simulink subsystem "bh_COMPONENT_3LINK_hand_Newton"  (R2022b)
settings: Solver=VariableStepAuto  StartTime=0.0  StopTime=10.0  RelTol=1e-3
undefined symbols (not defined in the file): IC, robo_params
settings Model: Creator=bhorton  LastModifiedBy=bhorton
settings SolverCC: AlgebraicLoopSolver=TrustRegion
settings DebuggingCC: UnconnectedInputMsg=warning  UnconnectedOutputMsg=warning  UnconnectedLineMsg=warning  SFMachineParentedDataDiag=warning
settings ModelReferenceCC: EnableRefExpFcnMdlSchedulingChecks=on
settings RTWCC: DLArmComputeVersion=19.05

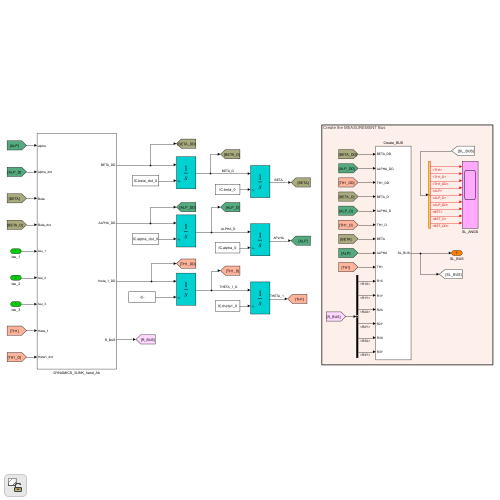
[thumbnail: Simulink's stored preview of the top-level diagram]
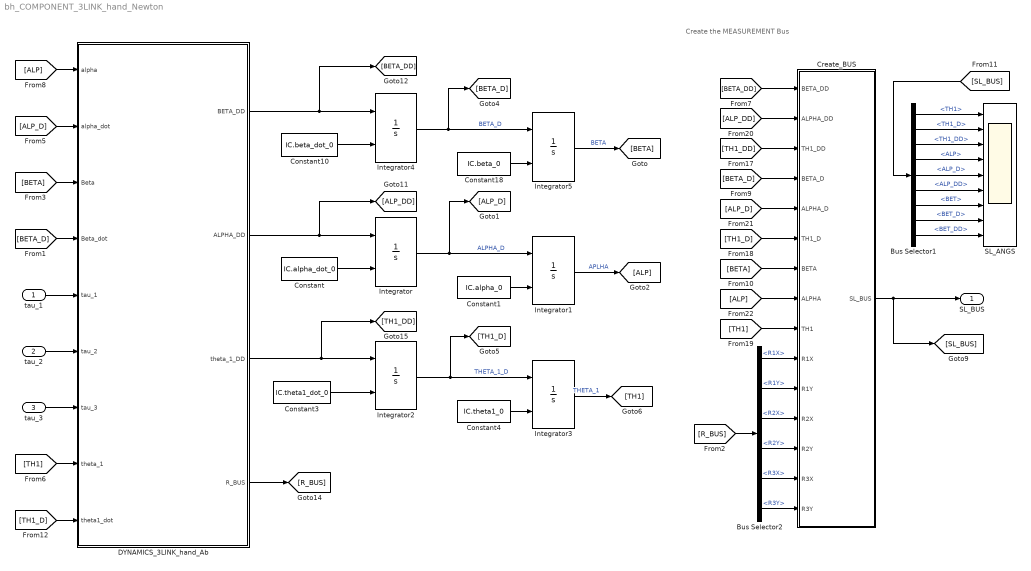
== system bh_COMPONENT_3LINK_hand_Newton ==
  note: Create the MEASUREMENT Bus
  tau_1 : Inport
  tau_2 : Inport  Port=2
  tau_3 : Inport  Port=3
  Bus Selector1 : BusSelector  OutputSignals=TH1,TH1_D,TH1_DD,ALP,ALP_D,ALP_DD,BET,BET_D,BET_DD
  Bus Selector2 : BusSelector  OutputSignals=R1X,R1Y,R2X,R2Y,R3X,R3Y
  Constant : Constant  Value=IC.alpha_dot_0
  Constant1 : Constant  Value=IC.alpha_0
  Constant10 : Constant  Value=IC.beta_dot_0
  Constant18 : Constant  Value=IC.beta_0
  Constant3 : Constant  Value=IC.theta1_dot_0
  Constant4 : Constant  Value=IC.theta1_0
  Create_BUS : Subsystem
  DYNAMICS_3LINK_hand_Ab : Subsystem
  Integrator{,1..5} (6 alike) : Integrator  InitialConditionSource=external
  SL_ANGS : Scope  NumInputPorts=9
  SL_BUS : Outport
  wires:
  Create_BUS/1(SL_BUS) -> SL_BUS/1, [SL_BUS]
  Bus Selector1/7 -> SL_ANGS/7  "<BET>"
  Bus Selector1/1 -> SL_ANGS/1  "<TH1>"
  [R_BUS] -> Bus Selector2/1
  [TH1] -> DYNAMICS_3LINK_hand_Ab/8(theta_1)
  DYNAMICS_3LINK_hand_Ab/4(R_BUS) -> [R_BUS]
  Bus Selector1/4 -> SL_ANGS/4  "<ALP>"
  [TH1_D] -> DYNAMICS_3LINK_hand_Ab/9(theta1_dot)
  tau_2/1 -> DYNAMICS_3LINK_hand_Ab/6(tau_2)
  Bus Selector1/3 -> SL_ANGS/3  "<TH1_DD>"
  Bus Selector2/1 -> Create_BUS/10(R1X)  "<R1X>"
  tau_3/1 -> DYNAMICS_3LINK_hand_Ab/7(tau_3)
  Bus Selector1/6 -> SL_ANGS/6  "<ALP_DD>"
  Bus Selector2/2 -> Create_BUS/11(R1Y)  "<R1Y>"
  DYNAMICS_3LINK_hand_Ab/2(ALPHA_DD) -> [ALP_DD], Integrator/1
  Constant1/1 -> Integrator1/2
  [BETA] -> DYNAMICS_3LINK_hand_Ab/3(Beta)
  tau_1/1 -> DYNAMICS_3LINK_hand_Ab/5(tau_1)
  [BETA_D] -> DYNAMICS_3LINK_hand_Ab/4(Beta_dot)
  [ALP] -> Create_BUS/8(ALPHA)
  [ALP] -> DYNAMICS_3LINK_hand_Ab/1(alpha)
  DYNAMICS_3LINK_hand_Ab/3(theta_1_DD) -> [TH1_DD], Integrator2/1
  [TH1_DD] -> Create_BUS/3(TH1_DD)
  [SL_BUS] -> Bus Selector1/1
  [BETA_D] -> Create_BUS/4(BETA_D)
  Bus Selector1/2 -> SL_ANGS/2  "<TH1_D>"
  Bus Selector1/5 -> SL_ANGS/5  "<ALP_D>"
  [BETA] -> Create_BUS/7(BETA)
  [ALP_DD] -> Create_BUS/2(ALPHA_DD)
  [BETA_DD] -> Create_BUS/1(BETA_DD)
  Bus Selector1/8 -> SL_ANGS/8  "<BET_D>"
  Constant18/1 -> Integrator5/2
  [ALP_D] -> Create_BUS/5(ALPHA_D)
  Integrator5/1 -> [BETA]  "BETA"
  [TH1] -> Create_BUS/9(TH1)
  DYNAMICS_3LINK_hand_Ab/1(BETA_DD) -> [BETA_DD], Integrator4/1
  Constant/1 -> Integrator/2
  Integrator2/1 -> [TH1_D], Integrator3/1  "THETA_1_D"
  Integrator4/1 -> [BETA_D], Integrator5/1  "BETA_D"
  Integrator1/1 -> [ALP]  "APLHA"
  Constant10/1 -> Integrator4/2
  Bus Selector1/9 -> SL_ANGS/9  "<BET_DD>"
  [TH1_D] -> Create_BUS/6(TH1_D)
  Integrator/1 -> [ALP_D], Integrator1/1  "ALPHA_D"
  [ALP_D] -> DYNAMICS_3LINK_hand_Ab/2(alpha_dot)
  Constant3/1 -> Integrator2/2
  Constant4/1 -> Integrator3/2
  Integrator3/1 -> [TH1]  "THETA_1"
  Bus Selector2/3 -> Create_BUS/12(R2X)  "<R2X>"
  Bus Selector2/4 -> Create_BUS/13(R2Y)  "<R2Y>"
  Bus Selector2/5 -> Create_BUS/14(R3X)  "<R3X>"
  Bus Selector2/6 -> Create_BUS/15(R3Y)  "<R3Y>"

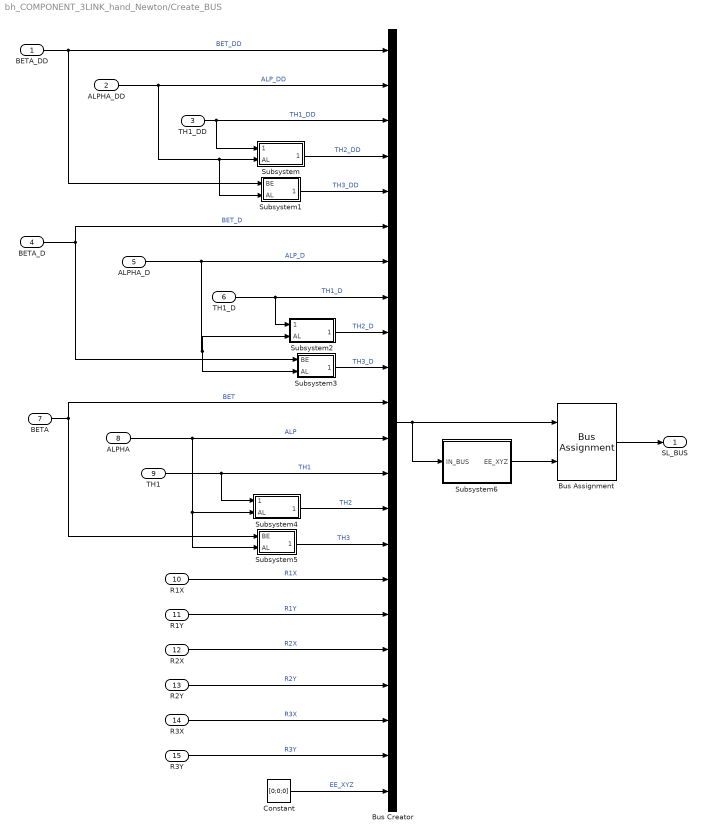
== system bh_COMPONENT_3LINK_hand_Newton/Create_BUS ==
  BETA_DD : Inport
  ALPHA_DD : Inport  Port=2
  TH1_DD : Inport  Port=3
  BETA_D : Inport  Port=4
  ALPHA_D : Inport  Port=5
  TH1_D : Inport  Port=6
  BETA : Inport  Port=7
  ALPHA : Inport  Port=8
  TH1 : Inport  Port=9
  R1X : Inport  Port=10
  R1Y : Inport  Port=11
  R2X : Inport  Port=12
  R2Y : Inport  Port=13
  R3X : Inport  Port=14
  R3Y : Inport  Port=15
  Bus Assignment : BusAssignment  AssignedSignals=EE_XYZ
  Bus Creator : BusCreator  Inputs=22
  Constant : Constant  Value=[0;0;0]
  Subsystem : Subsystem
  Subsystem1 : Subsystem
  Subsystem2 : Subsystem
  Subsystem3 : Subsystem
  Subsystem4 : Subsystem
  Subsystem5 : Subsystem
  Subsystem6 : Subsystem
  SL_BUS : Outport
  wires:
  BETA_DD/1 -> Subsystem1/1(BE), Bus Creator/1  "BET_DD"
  ALPHA_DD/1 -> Bus Creator/2, Subsystem1/2(AL), Subsystem/2(AL)  "ALP_DD"
  TH1_DD/1 -> Subsystem/1(TH_1), Bus Creator/3  "TH1_DD"
  Subsystem/1(TH_2) -> Bus Creator/4  "TH2_DD"
  Subsystem1/1(TH_3) -> Bus Creator/5  "TH3_DD"
  BETA_D/1 -> Subsystem3/1(BE), Bus Creator/6  "BET_D"
  ALPHA_D/1 -> Subsystem3/2(AL), Subsystem2/2(AL), Bus Creator/7  "ALP_D"
  TH1_D/1 -> Subsystem2/1(TH_1), Bus Creator/8  "TH1_D"
  Subsystem2/1(TH_2) -> Bus Creator/9  "TH2_D"
  Subsystem3/1(TH_3) -> Bus Creator/10  "TH3_D"
  BETA/1 -> Subsystem5/1(BE), Bus Creator/11  "BET"
  ALPHA/1 -> Subsystem5/2(AL), Subsystem4/2(AL), Bus Creator/12  "ALP"
  TH1/1 -> Subsystem4/1(TH_1), Bus Creator/13  "TH1"
  Subsystem4/1(TH_2) -> Bus Creator/14  "TH2"
  Subsystem5/1(TH_3) -> Bus Creator/15  "TH3"
  R1X/1 -> Bus Creator/16  "R1X"
  R1Y/1 -> Bus Creator/17  "R1Y"
  R2X/1 -> Bus Creator/18  "R2X"
  R2Y/1 -> Bus Creator/19  "R2Y"
  R3X/1 -> Bus Creator/20  "R3X"
  R3Y/1 -> Bus Creator/21  "R3Y"
  Constant/1 -> Bus Creator/22  "EE_XYZ"
  Bus Creator/1 -> Subsystem6/1(IN_BUS), Bus Assignment/1
  Subsystem6/1(EE_XYZ) -> Bus Assignment/2
  Bus Assignment/1 -> SL_BUS/1

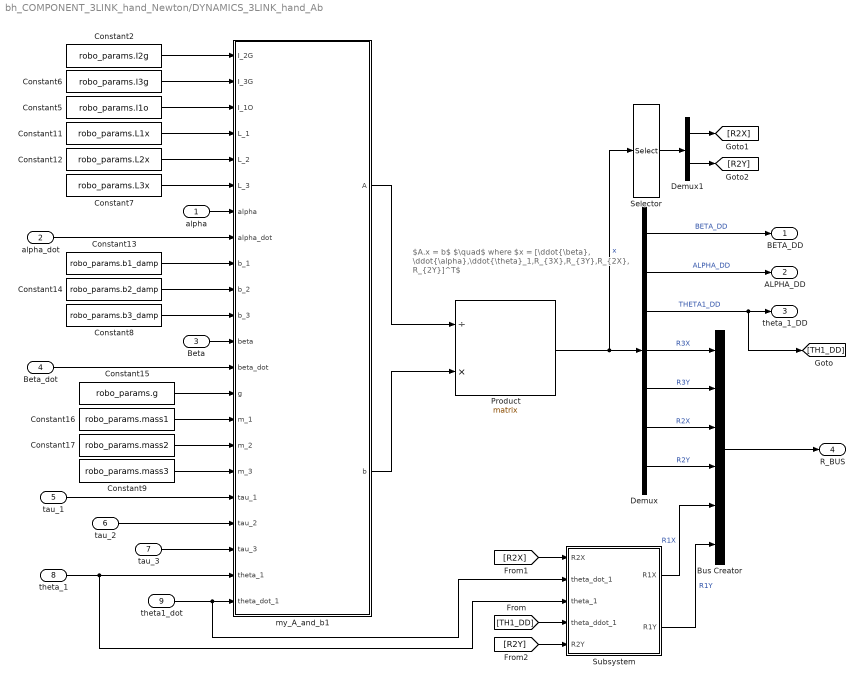
== system bh_COMPONENT_3LINK_hand_Newton/DYNAMICS_3LINK_hand_Ab ==
  note: $A.x = b$ $\quad$ where
      |
      | $x = [\ddot{\beta}, \ddot{\alpha},\ddot{\theta}_1,R_{3X},R_{3Y},R_{2X}, R_{2Y}]^T$
  alpha : Inport
  alpha_dot : Inport  Port=2
  Beta : Inport  Port=3
  Beta_dot : Inport  Port=4
  tau_1 : Inport  Port=5
  tau_2 : Inport  Port=6
  tau_3 : Inport  Port=7
  theta_1 : Inport  Port=8
  theta1_dot : Inport  Port=9
  Bus Creator : BusCreator  Inputs=6
  Constant11 : Constant  Value=robo_params.L1x
  Constant12 : Constant  Value=robo_params.L2x
  Constant13 : Constant  Value=robo_params.b1_damp
  Constant14 : Constant  Value=robo_params.b2_damp
  Constant15 : Constant  Value=robo_params.g
  Constant16 : Constant  Value=robo_params.mass1
  Constant17 : Constant  Value=robo_params.mass2
  Constant2 : Constant  Value=robo_params.I2g
  Constant5 : Constant  Value=robo_params.I1o
  Constant6 : Constant  Value=robo_params.I3g
  Constant7 : Constant  Value=robo_params.L3x
  Constant8 : Constant  Value=robo_params.b3_damp
  Constant9 : Constant  Value=robo_params.mass3
  Demux : Demux  Outputs=7
  Demux1 : Demux  Outputs=2
  Product : Product  Inputs=/*  Multiplication=Matrix(*)
  Selector : Selector  InputPortWidth=7  IndexOptions=Index vector (dialog)  Indices=[6 7]  OutputSizes=1
  Subsystem : Subsystem
  my_A_and_b1 : MATLAB Function  TreatAsAtomicUnit=on
  BETA_DD : Outport
  ALPHA_DD : Outport  Port=2
  theta_1_DD : Outport  Port=3
  R_BUS : Outport  Port=4
  wires:
  Bus Creator/1 -> R_BUS/1
  tau_1/1 -> my_A_and_b1/18(tau_1)
  Demux/2 -> ALPHA_DD/1  "ALPHA_DD"
  Subsystem/2(R1Y) -> Bus Creator/6  "R1Y"
  Demux/4 -> Bus Creator/1  "R3X"
  Constant14/1 -> my_A_and_b1/10(b_2)
  Demux/7 -> Bus Creator/4  "R2Y"
  Demux/1 -> BETA_DD/1  "BETA_DD"
  Subsystem/1(R1X) -> Bus Creator/5  "R1X"
  Constant9/1 -> my_A_and_b1/17(m_3)
  [R2Y] -> Subsystem/5(R2Y)
  Product/1 -> Demux/1, Selector/1  "x"
  alpha/1 -> my_A_and_b1/7(alpha)
  Constant5/1 -> my_A_and_b1/3(I_1O)
  Constant2/1 -> my_A_and_b1/1(I_2G)
  Constant12/1 -> my_A_and_b1/5(L_2)
  theta_1/1 -> my_A_and_b1/21(theta_1), Subsystem/3(theta_1)
  [TH1_DD] -> Subsystem/4(theta_ddot_1)
  Constant15/1 -> my_A_and_b1/14(g)
  Constant13/1 -> my_A_and_b1/9(b_1)
  alpha_dot/1 -> my_A_and_b1/8(alpha_dot)
  Demux/3 -> theta_1_DD/1, [TH1_DD]  "THETA1_DD"
  my_A_and_b1/1(A) -> Product/1
  tau_3/1 -> my_A_and_b1/20(tau_3)
  tau_2/1 -> my_A_and_b1/19(tau_2)
  Constant17/1 -> my_A_and_b1/16(m_2)
  [R2X] -> Subsystem/1(R2X)
  Demux/6 -> Bus Creator/3  "R2X"
  Constant6/1 -> my_A_and_b1/2(I_3G)
  Demux1/2 -> [R2Y]
  Demux/5 -> Bus Creator/2  "R3Y"
  my_A_and_b1/2(b) -> Product/2
  Demux1/1 -> [R2X]
  Beta/1 -> my_A_and_b1/12(beta)
  theta1_dot/1 -> my_A_and_b1/22(theta_dot_1), Subsystem/2(theta_dot_1)
  Beta_dot/1 -> my_A_and_b1/13(beta_dot)
  Constant11/1 -> my_A_and_b1/4(L_1)
  Selector/1 -> Demux1/1
  Constant7/1 -> my_A_and_b1/6(L_3)
  Constant8/1 -> my_A_and_b1/11(b_3)
  Constant16/1 -> my_A_and_b1/15(m_1)

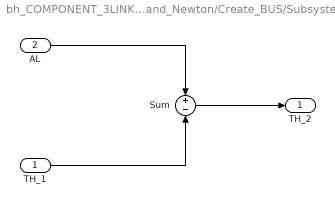
== system bh_COMPONENT_3LINK_hand_Newton/Create_BUS/Subsystem ==
  TH_1 : Inport
  AL : Inport  Port=2
  Sum : Sum  Inputs=+|-
  TH_2 : Outport
  wires:
  Sum/1 -> TH_2/1
  AL/1 -> Sum/1
  TH_1/1 -> Sum/2

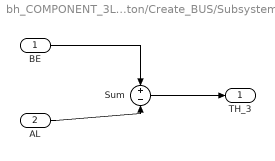
== system bh_COMPONENT_3LINK_hand_Newton/Create_BUS/Subsystem1 ==
  BE : Inport
  AL : Inport  Port=2
  Sum : Sum  Inputs=+|-
  TH_3 : Outport
  wires:
  BE/1 -> Sum/1
  AL/1 -> Sum/2
  Sum/1 -> TH_3/1

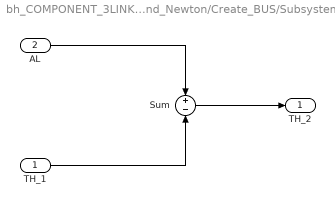
== system bh_COMPONENT_3LINK_hand_Newton/Create_BUS/Subsystem2 ==
  TH_1 : Inport
  AL : Inport  Port=2
  Sum : Sum  Inputs=+|-
  TH_2 : Outport
  wires:
  Sum/1 -> TH_2/1
  AL/1 -> Sum/1
  TH_1/1 -> Sum/2

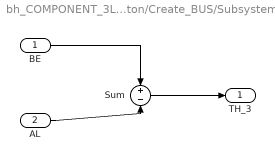
== system bh_COMPONENT_3LINK_hand_Newton/Create_BUS/Subsystem3 ==
  BE : Inport
  AL : Inport  Port=2
  Sum : Sum  Inputs=+|-
  TH_3 : Outport
  wires:
  BE/1 -> Sum/1
  AL/1 -> Sum/2
  Sum/1 -> TH_3/1

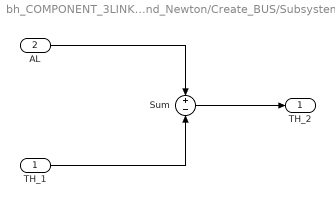
== system bh_COMPONENT_3LINK_hand_Newton/Create_BUS/Subsystem4 ==
  TH_1 : Inport
  AL : Inport  Port=2
  Sum : Sum  Inputs=+|-
  TH_2 : Outport
  wires:
  Sum/1 -> TH_2/1
  AL/1 -> Sum/1
  TH_1/1 -> Sum/2

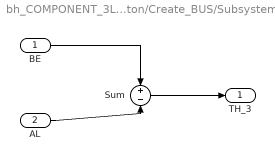
== system bh_COMPONENT_3LINK_hand_Newton/Create_BUS/Subsystem5 ==
  BE : Inport
  AL : Inport  Port=2
  Sum : Sum  Inputs=+|-
  TH_3 : Outport
  wires:
  BE/1 -> Sum/1
  AL/1 -> Sum/2
  Sum/1 -> TH_3/1

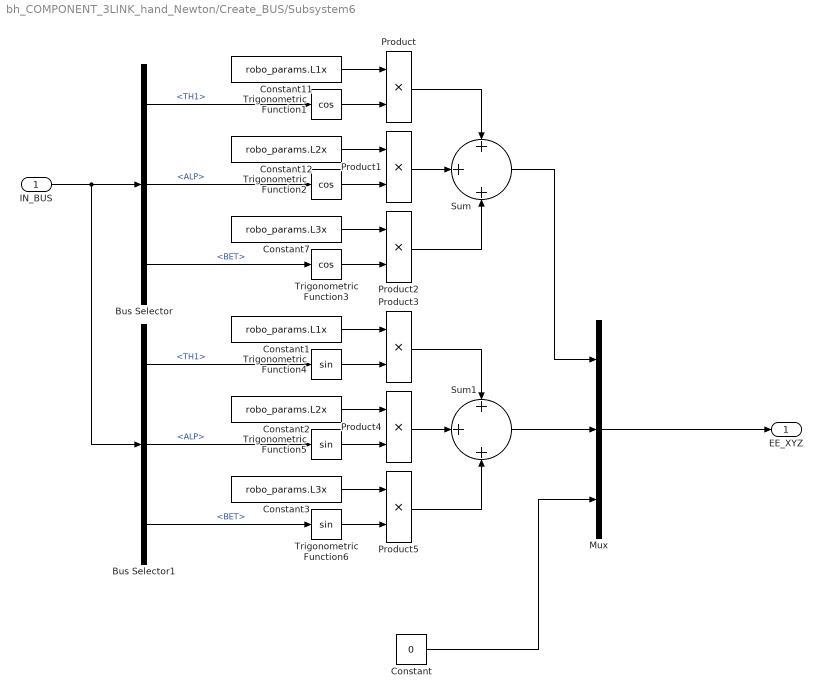
== system bh_COMPONENT_3LINK_hand_Newton/Create_BUS/Subsystem6 ==
  IN_BUS : Inport
  Bus Selector : BusSelector  OutputSignals=TH1,ALP,BET
  Bus Selector1 : BusSelector  OutputSignals=TH1,ALP,BET
  Constant : Constant  Value=0
  Constant1 : Constant  Value=robo_params.L1x
  Constant11 : Constant  Value=robo_params.L1x
  Constant12 : Constant  Value=robo_params.L2x
  Constant2 : Constant  Value=robo_params.L2x
  Constant3 : Constant  Value=robo_params.L3x
  Constant7 : Constant  Value=robo_params.L3x
  Mux : Mux  Inputs=3
  Product{,1..5} (6 alike) : Product
  Sum : Sum  Inputs=+|+|+
  Sum1 : Sum  Inputs=+|+|+
  Trigonometric Function1 : Trigonometry  Operator=cos
  Trigonometric Function2 : Trigonometry  Operator=cos
  Trigonometric Function3 : Trigonometry  Operator=cos
  Trigonometric Function4 : Trigonometry
  Trigonometric Function5 : Trigonometry
  Trigonometric Function6 : Trigonometry
  EE_XYZ : Outport
  wires:
  Bus Selector/1 -> Trigonometric Function1/1  "<TH1>"
  Bus Selector/2 -> Trigonometric Function2/1  "<ALP>"
  Bus Selector/3 -> Trigonometric Function3/1  "<BET>"
  Trigonometric Function1/1 -> Product/2
  Constant11/1 -> Product/1
  Trigonometric Function2/1 -> Product1/2
  Constant12/1 -> Product1/1
  Trigonometric Function3/1 -> Product2/2
  Constant7/1 -> Product2/1
  Product1/1 -> Sum/2
  Product/1 -> Sum/1
  Product2/1 -> Sum/3
  Bus Selector1/3 -> Trigonometric Function6/1  "<BET>"
  Bus Selector1/2 -> Trigonometric Function5/1  "<ALP>"
  Constant1/1 -> Product3/1
  IN_BUS/1 -> Bus Selector1/1, Bus Selector/1
  Bus Selector1/1 -> Trigonometric Function4/1  "<TH1>"
  Constant3/1 -> Product5/1
  Product5/1 -> Sum1/3
  Trigonometric Function6/1 -> Product5/2
  Trigonometric Function4/1 -> Product3/2
  Product3/1 -> Sum1/1
  Trigonometric Function5/1 -> Product4/2
  Constant2/1 -> Product4/1
  Product4/1 -> Sum1/2
  Sum/1 -> Mux/1
  Constant/1 -> Mux/3
  Sum1/1 -> Mux/2
  Mux/1 -> EE_XYZ/1

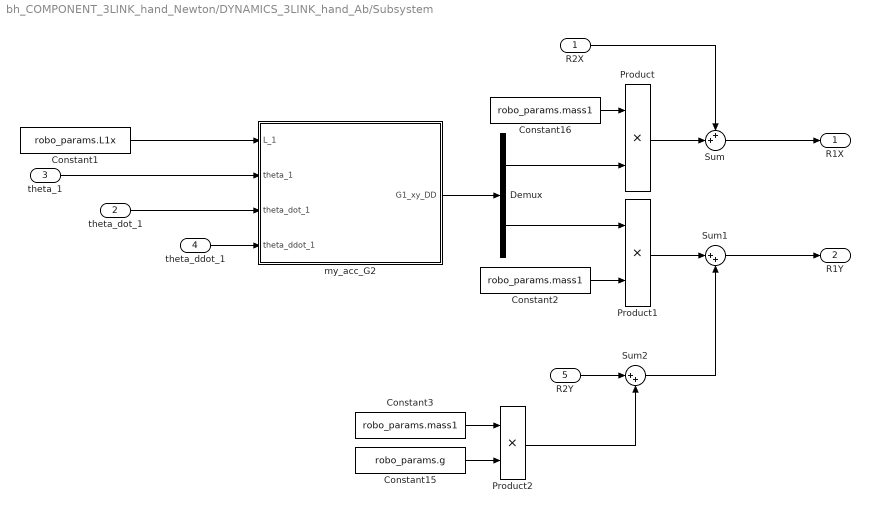
== system bh_COMPONENT_3LINK_hand_Newton/DYNAMICS_3LINK_hand_Ab/Subsystem ==
  R2X : Inport
  theta_dot_1 : Inport  Port=2
  theta_1 : Inport  Port=3
  theta_ddot_1 : Inport  Port=4
  R2Y : Inport  Port=5
  Constant1 : Constant  Value=robo_params.L1x
  Constant15 : Constant  Value=robo_params.g
  Constant16 : Constant  Value=robo_params.mass1
  Constant2 : Constant  Value=robo_params.mass1
  Constant3 : Constant  Value=robo_params.mass1
  Demux : Demux  Outputs=2
  Product : Product
  Product1 : Product
  Product2 : Product
  Sum : Sum  Inputs=++|
  Sum1 : Sum  Inputs=|++
  Sum2 : Sum  Inputs=|++
  my_acc_G2 : MATLAB Function  TreatAsAtomicUnit=on
  R1X : Outport
  R1Y : Outport  Port=2
  wires:
  R2Y/1 -> Sum2/1
  R2X/1 -> Sum/1
  Product2/1 -> Sum2/2
  Constant15/1 -> Product2/2
  Constant3/1 -> Product2/1
  Sum/1 -> R1X/1
  Sum1/1 -> R1Y/1
  Sum2/1 -> Sum1/2
  Product1/1 -> Sum1/1
  Constant2/1 -> Product1/2
  Demux/2 -> Product1/1
  Product/1 -> Sum/2
  Constant16/1 -> Product/1
  Demux/1 -> Product/2
  my_acc_G2/1(G1_xy_DD) -> Demux/1
  theta_dot_1/1 -> my_acc_G2/3(theta_dot_1)
  Constant1/1 -> my_acc_G2/1(L_1)
  theta_1/1 -> my_acc_G2/2(theta_1)
  theta_ddot_1/1 -> my_acc_G2/4(theta_ddot_1)

== matlab function bh_COMPONENT_3LINK_hand_Newton/DYNAMICS_3LINK_hand_Ab/my_A_and_b1 ==
  data: I_2G input; A output; I_3G input; I_1O input; L_1 input; L_2 input; L_3 input; alpha input; alpha_dot input; b_1 input; b_2 input; b_3 input; beta input; beta_dot input; g input; m_1 input; m_2 input; m_3 input; tau_1 input; tau_2 input; tau_3 input; theta_1 input; theta_dot_1 input; b output
function [A,b] = my_A_and_b(I_2G,I_3G,I_1O,L_1,L_2,L_3,alpha,alpha_dot,b_1,b_2,b_3,beta,beta_dot,g,m_1,m_2,m_3,tau_1,tau_2,tau_3,theta_1,theta_dot_1)
%#codegen

%    This function was generated by the Symbolic Math Toolbox version 9.2.
%    28-Oct-2022 10:28:51

A = reshape([L_3.*m_3.*sin(beta).*(-1.0./2.0),(L_3.*m_3.*cos(beta))./2.0,I_3G,0.0,0.0,0.0,0.0,-L_2.*m_3.*sin(alpha),L_2.*m_3.*cos(alpha),0.0,L_2.*m_2.*sin(alpha).*(-1.0./2.0),(L_2.*m_2.*cos(alpha))./2.0,I_2G,0.0,-L_1.*m_3.*sin(theta_1),L_1.*m_3.*cos(theta_1),0.0,-L_1.*m_2.*sin(theta_1),L_1.*m_2.*cos(theta_1),0.0,I_1O,-1.0,0.0,L_3.*sin(beta).*(-1.0./2.0),1.0,0.0,L_2.*sin(alpha).*(-1.0./2.0),0.0,0.0,-1.0,(L_3.*cos(beta))./2.0,0.0,1.0,(L_2.*cos(alpha))./2.0,0.0,0.0,0.0,0.0,-1.0,0.0,L_2.*sin(alpha).*(-1.0./2.0),-L_1.*sin(theta_1),0.0,0.0,0.0,0.0,-1.0,(L_2.*cos(alpha))./2.0,L_1.*cos(theta_1)],[7,7]);
if nargout > 1
    b = [m_3.*(L_2.*alpha_dot.^2.*cos(alpha)+(L_3.*beta_dot.^2.*cos(beta))./2.0+L_1.*theta_dot_1.^2.*cos(theta_1));m_3.*(L_2.*alpha_dot.^2.*sin(alpha)+(L_3.*beta_dot.^2.*sin(beta))./2.0+L_1.*theta_dot_1.^2.*sin(theta_1))-g.*m_3;tau_3+b_3.*(alpha_dot-beta_dot);m_2.*((L_2.*alpha_dot.^2.*cos(alpha))./2.0+L_1.*theta_dot_1.^2.*cos(theta_1));-g.*m_2+m_2.*((L_2.*alpha_dot.^2.*sin(alpha))./2.0+L_1.*theta_dot_1.^2.*sin(theta_1));tau_2-tau_3-b_3.*(alpha_dot-beta_dot)-b_2.*(alpha_dot-theta_dot_1);tau_1-tau_2-b_1.*theta_dot_1+b_2.*(alpha_dot-theta_dot_1)-(L_1.*g.*m_1.*cos(theta_1))./2.0];
end

== matlab function bh_COMPONENT_3LINK_hand_Newton/DYNAMICS_3LINK_hand_Ab/Subsystem/my_acc_G2 ==
  data: L_1 input; G1_xy_DD output; theta_1 input; theta_dot_1 input; theta_ddot_1 input
function G1_xy_DD = my_acc_G1(L_1,theta_1,theta_dot_1,theta_ddot_1)
%#codegen

%    This function was generated by the Symbolic Math Toolbox version 9.2.
%    28-Oct-2022 10:28:52

G1_xy_DD = [L_1.*theta_ddot_1.*sin(theta_1).*(-1.0./2.0)-(L_1.*theta_dot_1.^2.*cos(theta_1))./2.0;L_1.*theta_dot_1.^2.*sin(theta_1).*(-1.0./2.0)+(L_1.*theta_ddot_1.*cos(theta_1))./2.0];
